simulink model "zzz"  (R2016b)
settings: Solver=ode4  StartTime=0.0  StopTime=inf  FixedStep=0.002  RelTol=1e-3  EnableMultiTasking=on
undefined symbols (not defined in the file or in its folder): bit, mdaadlink6208, sigbuilder_block, Standard
libraries: slrtlib x19, simulink x15, slrtsoftinglib x11
(part 2 of 3)

== system zzz/guangaiquxian ==
  In1 : Inport
  Chart1 : Stateflow chart  TreatAsAtomicUnit=on
  Display : Display
  Fcn : Fcn  Expr=(3.76012963313985e-12)*u^16-(3.44037229998304e-10)*u^15+(1.39996774652558e-08)*u^14-(3.34309394387153e-07)*u^13+(5.21860519506510e-06)*u^12-(5.63398801585665e-05)*u^11+0.000435175092700704*u^10-0.00244274561068785*u^9+0.00982136561852038*u^8-0.0269377658736148*u^7+0.0514170009108526*u^6-0.103245210636221*u^5+0.431283025667506*u^4-2.79148222601809*u^3+0.0172306812740196*u^2-0.00241932536131526*u+600.000082443648
  Saturation : Saturate  UpperLimit=12  LowerLimit=0
  Saturation1 : Saturate  UpperLimit=600  LowerLimit=20
  Out1 : Outport
  wires:
  In1/1 -> Chart1/1(a)
  Chart1/1(t) -> Saturation/1
  Saturation/1 -> Fcn/1
  Fcn/1 -> Saturation1/1
  Saturation1/1 -> Display/1, Out1/1

== system zzz/jinjichuli ==
  tiaoshi : Inport
  fa : Inport  Port=2
  jiting : Inport  Port=3
  Enable : EnablePort  StatesWhenEnabling=reset
  Demux : Demux  Outputs=16
  Mux : Mux  Inputs=16
  jinjichuli : Stateflow chart  TreatAsAtomicUnit=on
  Out1 : Outport
  wires:
  tiaoshi/1 -> jinjichuli/1(tiaoshi)
  fa/1 -> Demux/1
  Demux/1 -> jinjichuli/2(fa11_1)
  Demux/2 -> jinjichuli/3(fa11_2)
  Demux/3 -> jinjichuli/4(fa11_5)
  Demux/4 -> jinjichuli/5(fa20)
  Demux/5 -> jinjichuli/6(fa16_1)
  Demux/6 -> jinjichuli/7(fa3)
  Demux/7 -> jinjichuli/8(fa21)
  Demux/12 -> jinjichuli/13(fa18_1)
  Demux/13 -> jinjichuli/14(fa18_2)
  jiting/1 -> jinjichuli/18(jiting)
  Demux/14 -> jinjichuli/15(fa18_3)
  Demux/15 -> jinjichuli/16(fa18_4)
  Demux/16 -> jinjichuli/17(fa_kgg)
  jinjichuli/1(diancifa11_1) -> Mux/1
  jinjichuli/2(diancifa11_2) -> Mux/2
  jinjichuli/3(diancifa11_5) -> Mux/3
  jinjichuli/4(diancifa20) -> Mux/4
  jinjichuli/5(diancifa16_1) -> Mux/5
  jinjichuli/6(diancifa3) -> Mux/6
  jinjichuli/7(diancifa21) -> Mux/7
  jinjichuli/12(bililiuliangfa18_1) -> Mux/12
  jinjichuli/13(bililiuliangfa18_2) -> Mux/13
  jinjichuli/14(bililiuliangfa18_3) -> Mux/14
  jinjichuli/15(bililiuliangfa18_4) -> Mux/15
  jinjichuli/16(kaiguangaifa) -> Mux/16
  Mux/1 -> Out1/1
  Demux/8 -> jinjichuli/9(suodingmingling)
  Demux/9 -> jinjichuli/10(jiesuomingling)
  Demux/10 -> jinjichuli/11(xuansongmingling)
  Demux/11 -> jinjichuli/12(xuanjinmingling)
  jinjichuli/8(suoding) -> Mux/8
  jinjichuli/9(jiesuo) -> Mux/9
  jinjichuli/10(xuansong) -> Mux/10
  jinjichuli/11(xuanjin) -> Mux/11

== system zzz/kaigaiquxian ==
  In1 : Inport
  Chart : Stateflow chart  TreatAsAtomicUnit=on
  Display : Display
  Fcn : Fcn  Expr=(3.76012794303783e-12)*u^16-(3.77787151438439e-10)*u^15+(1.70366716702520e-08)*u^14-(4.53918294904343e-07)*u^13+(7.91595568148143e-06)*u^12-(9.46991801150381e-05)*u^11+0.000795158956924619*u^10-0.00475883386986616*u^9+0.0207391801532158*u^8-0.0673081776269616*u^7+0.155366359479885*u^6-0.201490925155371*u^5-0.0768516231318135*u^4+2.18034933328387*u^3+0.0584293012534094*u^2-0.00654372848246011*u+20.0002376678902
  Saturation : Saturate  UpperLimit=12  LowerLimit=0
  Saturation1 : Saturate  UpperLimit=600  LowerLimit=20
  Out1 : Outport
  wires:
  In1/1 -> Chart/1(a)
  Saturation/1 -> Fcn/1
  Chart/1(t) -> Saturation/1
  Fcn/1 -> Saturation1/1
  Saturation1/1 -> Display/1, Out1/1

== system zzz/tiaoshifa ==
  Mux3 : Mux  Inputs=16
  fa11_1 : Constant  Value=0
      settings: OpenFcn=|
      | if get_param(gcb,'value')=='1',
      | set_param(gcb,'value','0');
      | else
      | set_param(gcb,'value','1');end
  fa11_2 : Constant  Value=0
      settings: OpenFcn=|
      | if get_param(gcb,'value')=='1',
      | set_param(gcb,'value','0');
      | else
      | set_param(gcb,'value','1');end
  fa11_5 : Constant  Value=0
      settings: OpenFcn=|
      | if get_param(gcb,'value')=='1',
      | set_param(gcb,'value','0');
      | else
      | set_param(gcb,'value','1');end
  fa16_1 : Constant  Value=0
      settings: OpenFcn=|
      | if get_param(gcb,'value')=='1',
      | set_param(gcb,'value','0');
      | else
      | set_param(gcb,'value','1');end
  fa18_{1..4} (4 alike) : Constant  Value=0
  fa20 : Constant  Value=0
      settings: OpenFcn=|
      | if get_param(gcb,'value')=='1',
      | set_param(gcb,'value','0');
      | else
      | set_param(gcb,'value','1');end
  fa21 : Constant  Value=0
      settings: OpenFcn=|
      | if get_param(gcb,'value')=='1',
      | set_param(gcb,'value','0');
      | else
      | set_param(gcb,'value','1');end
  fa3 : Constant  Value=0
      settings: OpenFcn=|
      | if get_param(gcb,'value')=='1',
      | set_param(gcb,'value','0');
      | else
      | set_param(gcb,'value','1');end
  fa_kgg : Constant  Value=0
  jiesuomingling : Constant  Value=0
      settings: OpenFcn=|
      | if get_param(gcb,'value')=='1',
      | set_param(gcb,'value','0');
      | else
      | set_param(gcb,'value','1');end
  suodingmingling : Constant  Value=0
      settings: OpenFcn=|
      | if get_param(gcb,'value')=='1',
      | set_param(gcb,'value','0');
      | else
      | set_param(gcb,'value','1');end
  xuanjinmingling : Constant  Value=0
      settings: OpenFcn=|
      | if get_param(gcb,'value')=='1',
      | set_param(gcb,'value','0');
      | else
      | set_param(gcb,'value','1');end
  xuansongmingling : Constant  Value=0
      settings: OpenFcn=|
      | if get_param(gcb,'value')=='1',
      | set_param(gcb,'value','0');
      | else
      | set_param(gcb,'value','1');end
  Out1 : Outport
  wires:
  fa11_5/1 -> Mux3/3
  fa20/1 -> Mux3/4
  jiesuomingling/1 -> Mux3/11
  xuanjinmingling/1 -> Mux3/9
  fa_kgg/1 -> Mux3/16
  fa11_2/1 -> Mux3/2
  fa11_1/1 -> Mux3/1
  fa16_1/1 -> Mux3/5
  xuansongmingling/1 -> Mux3/8
  fa21/1 -> Mux3/7
  suodingmingling/1 -> Mux3/10
  fa3/1 -> Mux3/6
  Mux3/1 -> Out1/1
  fa18_1/1 -> Mux3/12
  fa18_2/1 -> Mux3/13
  fa18_3/1 -> Mux3/14
  fa18_4/1 -> Mux3/15

== system zzz/Subsystem2/husuo ==
  In1 : Inport
  In2 : Inport  Port=2
  Constant : Constant  Value=0
  Constant2 : Constant  Value=0
  Memory : Memory
  Memory1 : Memory
  Switch : Switch  Criteria=u2 > Threshold  Threshold=0.5
  Switch2 : Switch  Criteria=u2 > Threshold  Threshold=0.5
  Out1 : Outport
  Out2 : Outport  Port=2
  wires:
  Memory/1 -> Switch/2
  Memory1/1 -> Switch2/2
  In1/1 -> Switch/3
  In2/1 -> Switch2/3
  Constant2/1 -> Switch2/1
  Switch/1 -> Memory1/1, Out1/1
  Constant/1 -> Switch/1
  Switch2/1 -> Out2/1, Memory/1

== system zzz/Subsystem2/husuo1 ==
  In1 : Inport
  In2 : Inport  Port=2
  Constant : Constant  Value=0
  Constant2 : Constant  Value=0
  Memory : Memory
  Memory1 : Memory
  Switch : Switch  Criteria=u2 > Threshold  Threshold=0.5
  Switch2 : Switch  Criteria=u2 > Threshold  Threshold=0.5
  Out1 : Outport
  Out2 : Outport  Port=2
  wires:
  Switch2/1 -> Memory/1, Out2/1
  Constant/1 -> Switch/1
  Switch/1 -> Out1/1, Memory1/1
  Constant2/1 -> Switch2/1
  In2/1 -> Switch2/3
  In1/1 -> Switch/3
  Memory1/1 -> Switch2/2
  Memory/1 -> Switch/2

== system zzz/Subsystem2/husuo2 ==
  In1 : Inport
  In2 : Inport  Port=2
  Constant : Constant  Value=0
  Constant2 : Constant  Value=0
  Memory : Memory
  Memory1 : Memory
  Switch : Switch  Criteria=u2 > Threshold  Threshold=0.5
  Switch2 : Switch  Criteria=u2 > Threshold  Threshold=0.5
  Out1 : Outport
  Out2 : Outport  Port=2
  wires:
  Memory/1 -> Switch/2
  Memory1/1 -> Switch2/2
  In1/1 -> Switch/3
  In2/1 -> Switch2/3
  Constant2/1 -> Switch2/1
  Switch/1 -> Memory1/1, Out1/1
  Constant/1 -> Switch/1
  Switch2/1 -> Out2/1, Memory/1

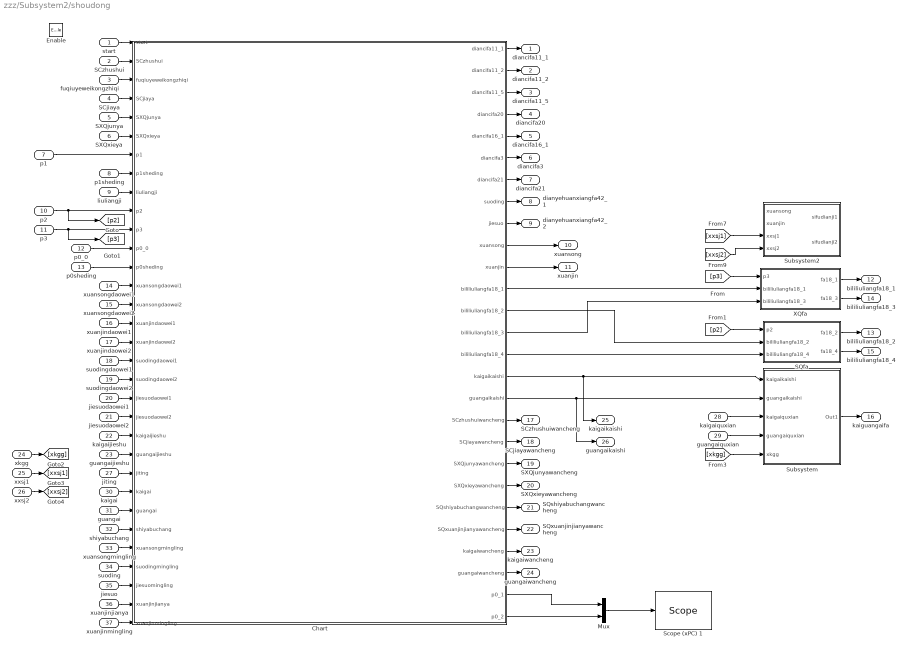
== system zzz/Subsystem2/shoudong ==
  start : Inport
  SCzhushui : Inport  Port=2
  fuqiuyeweikongzhiqi : Inport  Port=3
  SCjiaya : Inport  Port=4
  SXQjunya : Inport  Port=5
  SXQxieya : Inport  Port=6
  p1 : Inport  Port=7
  p1sheding : Inport  Port=8
  liuliangji : Inport  Port=9
  p2 : Inport  Port=10
  p3 : Inport  Port=11
  p0_0 : Inport  Port=12
  p0sheding : Inport  Port=13
  xuansongdaowei1 : Inport  Port=14
  xuansongdaowei2 : Inport  Port=15
  xuanjindaowei1 : Inport  Port=16
  xuanjindaowei2 : Inport  Port=17
  suodingdaowei1 : Inport  Port=18
  suodingdaowei2 : Inport  Port=19
  jiesuodaowei1 : Inport  Port=20
  jiesuodaowei2 : Inport  Port=21
  kaigaijieshu : Inport  Port=22
  guangaijieshu : Inport  Port=23
  xkgg : Inport  Port=24
  xxsj1 : Inport  Port=25
  xxsj2 : Inport  Port=26
  jiting : Inport  Port=27
  kaigaiquxian : Inport  Port=28
  guangaiquxian : Inport  Port=29
  kaigai : Inport  Port=30
  guangai : Inport  Port=31
  shiyabuchang : Inport  Port=32
  xuansongmingling : Inport  Port=33
  suoding : Inport  Port=34
  jiesuo : Inport  Port=35
  xuanjinjianya : Inport  Port=36
  xuanjinmingling : Inport  Port=37
  Enable : EnablePort
  Chart : Stateflow chart  TreatAsAtomicUnit=on
  Mux : Mux  Inputs=2
  SQfa : Subsystem
  Scope (xPC) 1 : slrtlib/Displays and Logging/Scope   scopeno=5  scopetype=Target  autostart=on  viewmode=Numerical  formatstr='%15.6f'  grid=on  ylimits=[0,0]  nosamples=250  noprepostsamples=0  interleave=1  triggermode=FreeRun  triggersignal=1  trigsignalfromport=off  triggerlevel=0.0  triggerslope=Either  triggerscope=1  triggersample=0  filename=data.dat  mode=Lazy  writesize=512  autorestart=off  dynamicfilemode=off  maxwritefilesize=512*1024^2
  Subsystem : Subsystem
  Subsystem2 : Subsystem
  XQfa : Subsystem
  diancifa11_1 : Outport
  diancifa11_2 : Outport  Port=2
  diancifa11_5 : Outport  Port=3
  diancifa20 : Outport  Port=4
  diancifa16_1 : Outport  Port=5
  diancifa3 : Outport  Port=6
  diancifa21 : Outport  Port=7
  dianyehuanxiangfa42_1 : Outport  Port=8
  dianyehuanxiangfa42_2 : Outport  Port=9
  xuansong : Outport  Port=10
  xuanjin : Outport  Port=11
  bililiuliangfa18_1 : Outport  Port=12
  bililiuliangfa18_2 : Outport  Port=13
  bililiuliangfa18_3 : Outport  Port=14
  bililiuliangfa18_4 : Outport  Port=15
  kaiguangaifa : Outport  Port=16
  SCzhushuiwancheng : Outport  Port=17
  SCjiayawancheng : Outport  Port=18
  SXQjunyawancheng : Outport  Port=19
  SXQxieyawancheng : Outport  Port=20
  SQshiyabuchangwancheng : Outport  Port=21
  SQxuanjinjianyawancheng : Outport  Port=22
  kaigaiwancheng : Outport  Port=23
  guangaiwancheng : Outport  Port=24
  kaigaikaishi : Outport  Port=25
  guangaikaishi : Outport  Port=26
  wires:
  jiting/1 -> Chart/24(jiting)
  xkgg/1 -> [xkgg]
  Chart/23(SQxuanjinjianyawancheng) -> SQxuanjinjianyawancheng/1
  Chart/22(SQshiyabuchangwancheng) -> SQshiyabuchangwancheng/1
  Chart/21(SXQxieyawancheng) -> SXQxieyawancheng/1
  Chart/20(SXQjunyawancheng) -> SXQjunyawancheng/1
  Chart/19(SCjiayawancheng) -> SCjiayawancheng/1
  Chart/18(SCzhushuiwancheng) -> SCzhushuiwancheng/1
  Chart/9(jiesuo) -> dianyehuanxiangfa42_2/1
  Chart/8(suoding) -> dianyehuanxiangfa42_1/1
  Chart/25(guangaiwancheng) -> guangaiwancheng/1
  guangaijieshu/1 -> Chart/23(guangaijieshu)
  Chart/24(kaigaiwancheng) -> kaigaiwancheng/1
  kaigaijieshu/1 -> Chart/22(kaigaijieshu)
  jiesuodaowei2/1 -> Chart/21(jiesuodaowei2)
  jiesuodaowei1/1 -> Chart/20(jiesuodaowei1)
  suodingdaowei2/1 -> Chart/19(suodingdaowei2)
  suodingdaowei1/1 -> Chart/18(suodingdaowei1)
  xuanjindaowei2/1 -> Chart/17(xuanjindaowei2)
  xuanjindaowei1/1 -> Chart/16(xuanjindaowei1)
  xuansongdaowei2/1 -> Chart/15(xuansongdaowei2)
  xuansongdaowei1/1 -> Chart/14(xuansongdaowei1)
  guangai/1 -> Chart/26(guangai)
  kaigai/1 -> Chart/25(kaigai)
  SQfa/2(fa18_4) -> bililiuliangfa18_4/1
  SQfa/1(fa18_2) -> bililiuliangfa18_2/1
  liuliangji/1 -> Chart/9(liuliangji)
  XQfa/2(fa18_3) -> bililiuliangfa18_3/1
  Chart/7(diancifa21) -> diancifa21/1
  XQfa/1(fa18_1) -> bililiuliangfa18_1/1
  Chart/6(diancifa3) -> diancifa3/1
  SXQxieya/1 -> Chart/6(SXQxieya)
  Chart/5(diancifa16_1) -> diancifa16_1/1
  SXQjunya/1 -> Chart/5(SXQjunya)
  Chart/4(diancifa20) -> diancifa20/1
  SCjiaya/1 -> Chart/4(SCjiaya)
  Chart/3(diancifa11_5) -> diancifa11_5/1
  fuqiuyeweikongzhiqi/1 -> Chart/3(fuqiuyeweikongzhiqi)
  Chart/2(diancifa11_2) -> diancifa11_2/1
  SCzhushui/1 -> Chart/2(SCzhushui)
  Chart/1(diancifa11_1) -> diancifa11_1/1
  start/1 -> Chart/1(start)
  p1/1 -> Chart/7(p1)
  [p2] -> SQfa/1(p2)
  [p3] -> XQfa/1(p3)
  p3/1 -> [p3], Chart/11(p3)
  p2/1 -> [p2], Chart/10(p2)
  p0_0/1 -> Chart/12(p0_0)
  p0sheding/1 -> Chart/13(p0sheding)
  p1sheding/1 -> Chart/8(p1sheding)
  Chart/15(bililiuliangfa18_4) -> SQfa/3(bililiuliangfa18_4)
  Chart/12(bililiuliangfa18_1) -> XQfa/2(bililiuliangfa18_1)
  Chart/13(bililiuliangfa18_2) -> SQfa/2(bililiuliangfa18_2)
  Chart/14(bililiuliangfa18_3) -> XQfa/3(bililiuliangfa18_3)
  shiyabuchang/1 -> Chart/27(shiyabuchang)
  xuansongmingling/1 -> Chart/28(xuansongmingling)
  suoding/1 -> Chart/29(suodingmingling)
  jiesuo/1 -> Chart/30(jiesuomingling)
  xuanjinjianya/1 -> Chart/31(xuanjinjianya)
  xuanjinmingling/1 -> Chart/32(xuanjinmingling)
  xxsj1/1 -> [xxsj1]
  xxsj2/1 -> [xxsj2]
  [xkgg] -> Subsystem/5(xkgg)
  Subsystem/1(Out1) -> kaiguangaifa/1
  [xxsj2] -> Subsystem2/4(xxsj2)
  [xxsj1] -> Subsystem2/3(xxsj1)
  Chart/10(xuansong) -> xuansong/1
  Chart/11(xuanjin) -> xuanjin/1
  Chart/26(p0_1) -> Mux/1
  Chart/27(p0_2) -> Mux/2
  Mux/1 -> Scope (xPC) 1/1
  Chart/16(kaigaikaishi) -> kaigaikaishi/1, Subsystem/1(kaigaikaishi)
  Chart/17(guangaikaishi) -> Subsystem/2(guangaikaishi), guangaikaishi/1
  guangaiquxian/1 -> Subsystem/4(guangaiquxian)
  kaigaiquxian/1 -> Subsystem/3(kaigaiquxian)

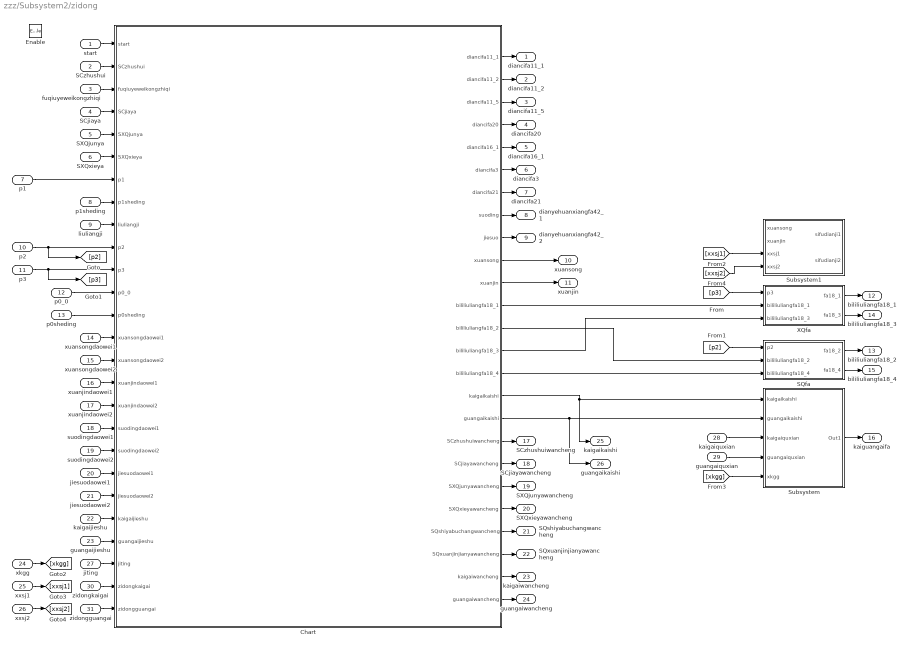
== system zzz/Subsystem2/zidong ==
  start : Inport
  SCzhushui : Inport  Port=2
  fuqiuyeweikongzhiqi : Inport  Port=3
  SCjiaya : Inport  Port=4
  SXQjunya : Inport  Port=5
  SXQxieya : Inport  Port=6
  p1 : Inport  Port=7
  p1sheding : Inport  Port=8
  liuliangji : Inport  Port=9
  p2 : Inport  Port=10
  p3 : Inport  Port=11
  p0_0 : Inport  Port=12
  p0sheding : Inport  Port=13
  xuansongdaowei1 : Inport  Port=14
  xuansongdaowei2 : Inport  Port=15
  xuanjindaowei1 : Inport  Port=16
  xuanjindaowei2 : Inport  Port=17
  suodingdaowei1 : Inport  Port=18
  suodingdaowei2 : Inport  Port=19
  jiesuodaowei1 : Inport  Port=20
  jiesuodaowei2 : Inport  Port=21
  kaigaijieshu : Inport  Port=22
  guangaijieshu : Inport  Port=23
  xkgg : Inport  Port=24
  xxsj1 : Inport  Port=25
  xxsj2 : Inport  Port=26
  jiting : Inport  Port=27
  kaigaiquxian : Inport  Port=28
  guangaiquxian : Inport  Port=29
  zidongkaigai : Inport  Port=30
  zidongguangai : Inport  Port=31
  Enable : EnablePort
  Chart : Stateflow chart  TreatAsAtomicUnit=on
  SQfa : Subsystem
  Subsystem : Subsystem
  Subsystem1 : Subsystem
  XQfa : Subsystem
  diancifa11_1 : Outport
  diancifa11_2 : Outport  Port=2
  diancifa11_5 : Outport  Port=3
  diancifa20 : Outport  Port=4
  diancifa16_1 : Outport  Port=5
  diancifa3 : Outport  Port=6
  diancifa21 : Outport  Port=7
  dianyehuanxiangfa42_1 : Outport  Port=8
  dianyehuanxiangfa42_2 : Outport  Port=9
  xuansong : Outport  Port=10
  xuanjin : Outport  Port=11
  bililiuliangfa18_1 : Outport  Port=12
  bililiuliangfa18_2 : Outport  Port=13
  bililiuliangfa18_3 : Outport  Port=14
  bililiuliangfa18_4 : Outport  Port=15
  kaiguangaifa : Outport  Port=16
  SCzhushuiwancheng : Outport  Port=17
  SCjiayawancheng : Outport  Port=18
  SXQjunyawancheng : Outport  Port=19
  SXQxieyawancheng : Outport  Port=20
  SQshiyabuchangwancheng : Outport  Port=21
  SQxuanjinjianyawancheng : Outport  Port=22
  kaigaiwancheng : Outport  Port=23
  guangaiwancheng : Outport  Port=24
  kaigaikaishi : Outport  Port=25
  guangaikaishi : Outport  Port=26
  wires:
  Chart/14(bililiuliangfa18_3) -> XQfa/3(bililiuliangfa18_3)
  Chart/13(bililiuliangfa18_2) -> SQfa/2(bililiuliangfa18_2)
  Chart/12(bililiuliangfa18_1) -> XQfa/2(bililiuliangfa18_1)
  Chart/15(bililiuliangfa18_4) -> SQfa/3(bililiuliangfa18_4)
  p1sheding/1 -> Chart/8(p1sheding)
  p0sheding/1 -> Chart/13(p0sheding)
  p0_0/1 -> Chart/12(p0_0)
  p2/1 -> Chart/10(p2), [p2]
  p3/1 -> Chart/11(p3), [p3]
  [p3] -> XQfa/1(p3)
  [p2] -> SQfa/1(p2)
  p1/1 -> Chart/7(p1)
  start/1 -> Chart/1(start)
  Chart/1(diancifa11_1) -> diancifa11_1/1
  SCzhushui/1 -> Chart/2(SCzhushui)
  Chart/2(diancifa11_2) -> diancifa11_2/1
  fuqiuyeweikongzhiqi/1 -> Chart/3(fuqiuyeweikongzhiqi)
  Chart/3(diancifa11_5) -> diancifa11_5/1
  SCjiaya/1 -> Chart/4(SCjiaya)
  Chart/4(diancifa20) -> diancifa20/1
  SXQjunya/1 -> Chart/5(SXQjunya)
  Chart/5(diancifa16_1) -> diancifa16_1/1
  SXQxieya/1 -> Chart/6(SXQxieya)
  Chart/6(diancifa3) -> diancifa3/1
  XQfa/1(fa18_1) -> bililiuliangfa18_1/1
  Chart/7(diancifa21) -> diancifa21/1
  XQfa/2(fa18_3) -> bililiuliangfa18_3/1
  liuliangji/1 -> Chart/9(liuliangji)
  SQfa/1(fa18_2) -> bililiuliangfa18_2/1
  SQfa/2(fa18_4) -> bililiuliangfa18_4/1
  zidongkaigai/1 -> Chart/25(zidongkaigai)
  zidongguangai/1 -> Chart/26(zidongguangai)
  xuansongdaowei1/1 -> Chart/14(xuansongdaowei1)
  xuansongdaowei2/1 -> Chart/15(xuansongdaowei2)
  xuanjindaowei1/1 -> Chart/16(xuanjindaowei1)
  xuanjindaowei2/1 -> Chart/17(xuanjindaowei2)
  suodingdaowei1/1 -> Chart/18(suodingdaowei1)
  suodingdaowei2/1 -> Chart/19(suodingdaowei2)
  jiesuodaowei1/1 -> Chart/20(jiesuodaowei1)
  jiesuodaowei2/1 -> Chart/21(jiesuodaowei2)
  kaigaijieshu/1 -> Chart/22(kaigaijieshu)
  Chart/24(kaigaiwancheng) -> kaigaiwancheng/1
  guangaijieshu/1 -> Chart/23(guangaijieshu)
  Chart/25(guangaiwancheng) -> guangaiwancheng/1
  Chart/8(suoding) -> dianyehuanxiangfa42_1/1
  Chart/9(jiesuo) -> dianyehuanxiangfa42_2/1
  Chart/18(SCzhushuiwancheng) -> SCzhushuiwancheng/1
  Chart/19(SCjiayawancheng) -> SCjiayawancheng/1
  Chart/20(SXQjunyawancheng) -> SXQjunyawancheng/1
  Chart/21(SXQxieyawancheng) -> SXQxieyawancheng/1
  Chart/22(SQshiyabuchangwancheng) -> SQshiyabuchangwancheng/1
  Chart/23(SQxuanjinjianyawancheng) -> SQxuanjinjianyawancheng/1
  xkgg/1 -> [xkgg]
  jiting/1 -> Chart/24(jiting)
  xxsj1/1 -> [xxsj1]
  xxsj2/1 -> [xxsj2]
  Chart/16(kaigaikaishi) -> kaigaikaishi/1, Subsystem/1(kaigaikaishi)
  Chart/17(guangaikaishi) -> guangaikaishi/1, Subsystem/2(guangaikaishi)
  [xkgg] -> Subsystem/5(xkgg)
  Subsystem/1(Out1) -> kaiguangaifa/1
  [xxsj2] -> Subsystem1/4(xxsj2)
  [xxsj1] -> Subsystem1/3(xxsj1)
  Chart/10(xuansong) -> xuansong/1
  Chart/11(xuanjin) -> xuanjin/1
  kaigaiquxian/1 -> Subsystem/3(kaigaiquxian)
  guangaiquxian/1 -> Subsystem/4(guangaiquxian)

== system zzz/chuanganqi/yalishangxiaxian ==
  In1 : Inport
  Compare To Constant{,2,4,6,8,10} (6 alike) : simulink/Logic and Bit Operations/Compare To Constant  relop=<=  const=0.1  OutDataTypeStr=boolean
  Compare To Constant{1,3,5,7,9,11} (6 alike) : simulink/Logic and Bit Operations/Compare To Constant  relop=>=  const=0.33  OutDataTypeStr=boolean
  Demux5 : Demux  Outputs=6
  Logical Operator : Logic  Operator=OR  Inputs=12  AllPortsSameDT=off  OutDataTypeStr=boolean
  Out1 : Outport
  wires:
  Demux5/2 -> Compare To Constant3/1, Compare To Constant2/1
  Demux5/6 -> Compare To Constant11/1, Compare To Constant10/1
  Compare To Constant/1 -> Logical Operator/1
  Demux5/4 -> Compare To Constant7/1, Compare To Constant6/1
  Compare To Constant8/1 -> Logical Operator/9
  Compare To Constant9/1 -> Logical Operator/10
  Compare To Constant4/1 -> Logical Operator/5
  Compare To Constant5/1 -> Logical Operator/6
  Compare To Constant2/1 -> Logical Operator/3
  Compare To Constant3/1 -> Logical Operator/4
  Compare To Constant6/1 -> Logical Operator/7
  Compare To Constant7/1 -> Logical Operator/8
  Compare To Constant11/1 -> Logical Operator/12
  Compare To Constant10/1 -> Logical Operator/11
  Demux5/3 -> Compare To Constant5/1, Compare To Constant4/1
  Demux5/1 -> Compare To Constant1/1, Compare To Constant/1
  Demux5/5 -> Compare To Constant9/1, Compare To Constant8/1
  In1/1 -> Demux5/1
  Compare To Constant1/1 -> Logical Operator/2
  Logical Operator/1 -> Out1/1

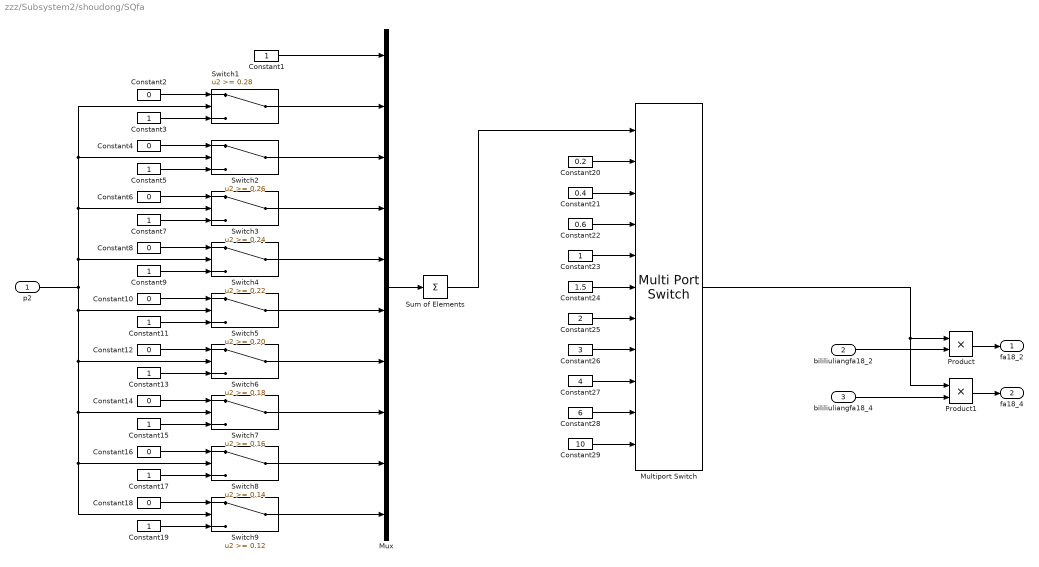
== system zzz/Subsystem2/shoudong/SQfa ==
  p2 : Inport
  bililiuliangfa18_2 : Inport  Port=2
  bililiuliangfa18_4 : Inport  Port=3
  Constant{1,3,5,7,9,11,13,15,17,19,23} (11 alike) : Constant
  Constant{2,4,6,8,10,12,14,16,18} (9 alike) : Constant  Value=0
  Constant20 : Constant  Value=0.2
  Constant21 : Constant  Value=0.4
  Constant22 : Constant  Value=0.6
  Constant24 : Constant  Value=1.5
  Constant25 : Constant  Value=2
  Constant26 : Constant  Value=3
  Constant27 : Constant  Value=4
  Constant28 : Constant  Value=6
  Constant29 : Constant  Value=10
  Multiport Switch : MultiPortSwitch  Inputs=10
  Mux : Mux  Inputs=10
  Product : Product  RndMeth=Zero
  Product1 : Product  RndMeth=Zero
  Sum of Elements : Sum  Inputs=+
  Switch1 : Switch  Threshold=0.28
  Switch2 : Switch  Threshold=0.26
  Switch3 : Switch  Threshold=0.24
  Switch4 : Switch  Threshold=0.22
  Switch5 : Switch  Threshold=0.20
  Switch6 : Switch  Threshold=0.18
  Switch7 : Switch  Threshold=0.16
  Switch8 : Switch  Threshold=0.14
  Switch9 : Switch  Threshold=0.12
  fa18_2 : Outport
  fa18_4 : Outport  Port=2
  wires:
  Constant2/1 -> Switch1/1
  Constant3/1 -> Switch1/3
  Constant4/1 -> Switch2/1
  Constant5/1 -> Switch2/3
  Constant6/1 -> Switch3/1
  Constant7/1 -> Switch3/3
  Constant8/1 -> Switch4/1
  Constant9/1 -> Switch4/3
  Constant10/1 -> Switch5/1
  Constant11/1 -> Switch5/3
  Constant12/1 -> Switch6/1
  Constant13/1 -> Switch6/3
  Constant14/1 -> Switch7/1
  Constant15/1 -> Switch7/3
  p2/1 -> Switch1/2, Switch2/2, Switch3/2, Switch4/2, Switch6/2, Switch7/2, Switch8/2, Switch9/2, Switch5/2
  Mux/1 -> Sum of Elements/1
  Sum of Elements/1 -> Multiport Switch/1
  Constant1/1 -> Mux/1
  Switch1/1 -> Mux/2
  Switch2/1 -> Mux/3
  Switch3/1 -> Mux/4
  Switch4/1 -> Mux/5
  Switch5/1 -> Mux/6
  Switch6/1 -> Mux/7
  Switch7/1 -> Mux/8
  Switch8/1 -> Mux/9
  Switch9/1 -> Mux/10
  Constant16/1 -> Switch8/1
  Constant17/1 -> Switch8/3
  Constant18/1 -> Switch9/1
  Constant19/1 -> Switch9/3
  Multiport Switch/1 -> Product/1, Product1/1
  Constant20/1 -> Multiport Switch/2
  Constant21/1 -> Multiport Switch/3
  Constant22/1 -> Multiport Switch/4
  Constant23/1 -> Multiport Switch/5
  Constant24/1 -> Multiport Switch/6
  Constant25/1 -> Multiport Switch/7
  Constant26/1 -> Multiport Switch/8
  Constant27/1 -> Multiport Switch/9
  Constant28/1 -> Multiport Switch/10
  Constant29/1 -> Multiport Switch/11
  bililiuliangfa18_2/1 -> Product/2
  bililiuliangfa18_4/1 -> Product1/2
  Product/1 -> fa18_2/1
  Product1/1 -> fa18_4/1

== system zzz/Subsystem2/shoudong/Subsystem ==
  kaigaikaishi : Inport
  guangaikaishi : Inport  Port=2
  kaigaiquxian : Inport  Port=3
  guangaiquxian : Inport  Port=4
  xkgg : Inport  Port=5
  Add1 : Sum
  Constant : Constant  Value=2
  Constant1 : Constant  Value=-0.05
  Display{,1..3} (4 alike) : Display
  Gain : Gain  Gain=0.1
  Gain1 : Gain  Gain=0.1
  Multiport Switch : MultiPortSwitch
  Product : Product
  Sum : Sum  Inputs=|+-
  Sum1 : Sum  Inputs=|+-
  Out1 : Outport
  wires:
  guangaikaishi/1 -> Product/1
  Constant/1 -> Product/2
  kaigaikaishi/1 -> Add1/1
  Product/1 -> Add1/2
  Add1/1 -> Multiport Switch/1
  Multiport Switch/1 -> Display2/1, Out1/1
  Sum/1 -> Gain/1
  Gain/1 -> Multiport Switch/2, Display1/1
  Sum1/1 -> Gain1/1
  Gain1/1 -> Display/1, Multiport Switch/3
  Constant1/1 -> Multiport Switch/4
  xkgg/1 -> Display3/1, Sum1/2, Sum/2
  kaigaiquxian/1 -> Sum/1
  guangaiquxian/1 -> Sum1/1

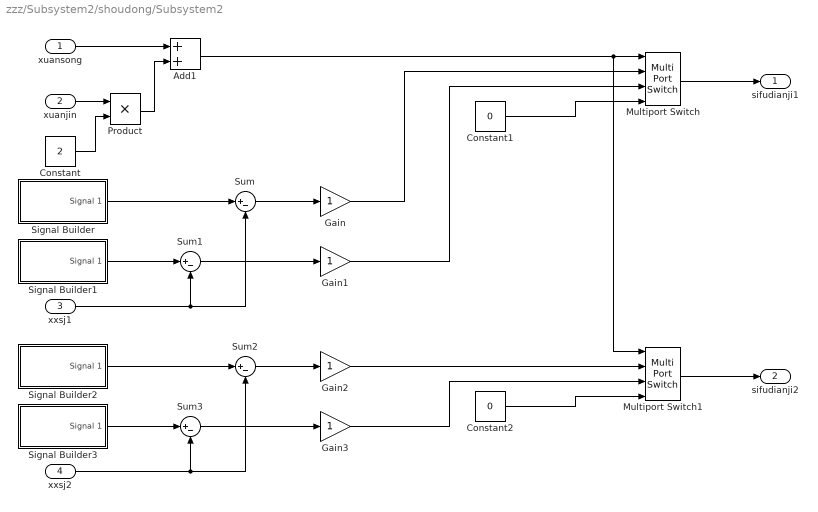
== system zzz/Subsystem2/shoudong/Subsystem2 ==
  xuansong : Inport
  xuanjin : Inport  Port=2
  xxsj1 : Inport  Port=3
  xxsj2 : Inport  Port=4
  Add1 : Sum
  Constant : Constant  Value=2
  Constant1 : Constant  Value=0
  Constant2 : Constant  Value=0
  Gain{,1..3} (4 alike) : Gain
  Multiport Switch : MultiPortSwitch
  Multiport Switch1 : MultiPortSwitch
  Product : Product
  Signal Builder : Subsystem  Tag=STV Subsys  LoadFcn=sigbuilder_block('load');  StartFcn=sigbuilder_block('start');  StopFcn=sigbuilder_block('stop');  ClipboardFcn=sigbuilder_block('clipboard');  mask(Sigbuilder block){tuvar=[0:10]}
      mask help: Simulink:masks:SigbuilderBlock_MD
      mask init:
      | if ~strcmp(get_param(bdroot(gcbh),'SimulationStatus'),'stopped') tuvar = sigbuilder_block('maskInit'); end
      settings: CopyFcn=sigbuilder_block('copy');  DeleteFcn=sigbuilder_block('delete');  ModelCloseFcn=sigbuilder_block('modelClose');  PreSaveFcn=sigbuilder_block('preSave');  PauseFcn=sigbuilder_block('pause');  ContinueFcn=sigbuilder_block('continue');  NameChangeFcn=sigbuilder_block('namechange');  OpenFcn=sigbuilder_block('open',[437.6 199.2 550.4 400 ]);  CloseFcn=sigbuilder_block('close');
      mask Display: plot(0, 0, 100, 100,[2, 2, 32, 32, 2], [68, 8, 8, 68, 68],[32, 2], [38, 38], [32, 19, 2],[53, 60, 44], [32, 17, 17, 2],[16, 16, 31, 31]);txt = getActiveGroup(gcbh);text(2, 100, txt,'verticalAlignment', 'top');
  Signal Builder1 : Subsystem  Tag=STV Subsys  LoadFcn=sigbuilder_block('load');  StartFcn=sigbuilder_block('start');  StopFcn=sigbuilder_block('stop');  ClipboardFcn=sigbuilder_block('clipboard');  mask(Sigbuilder block){tuvar=[0:10]}
      mask help: Simulink:masks:SigbuilderBlock_MD
      mask init:
      | if ~strcmp(get_param(bdroot(gcbh),'SimulationStatus'),'stopped') tuvar = sigbuilder_block('maskInit'); end
      settings: CopyFcn=sigbuilder_block('copy');  DeleteFcn=sigbuilder_block('delete');  ModelCloseFcn=sigbuilder_block('modelClose');  PreSaveFcn=sigbuilder_block('preSave');  PauseFcn=sigbuilder_block('pause');  ContinueFcn=sigbuilder_block('continue');  NameChangeFcn=sigbuilder_block('namechange');  OpenFcn=sigbuilder_block('open',[437.6 199.2 550.4 400 ]);  CloseFcn=sigbuilder_block('close');
      mask Display: plot(0, 0, 100, 100,[2, 2, 32, 32, 2], [68, 8, 8, 68, 68],[32, 2], [38, 38], [32, 19, 2],[53, 60, 44], [32, 17, 17, 2],[16, 16, 31, 31]);txt = getActiveGroup(gcbh);text(2, 100, txt,'verticalAlignment', 'top');
  Signal Builder2 : Subsystem  Tag=STV Subsys  LoadFcn=sigbuilder_block('load');  StartFcn=sigbuilder_block('start');  StopFcn=sigbuilder_block('stop');  ClipboardFcn=sigbuilder_block('clipboard');  mask(Sigbuilder block){tuvar=[0:10]}
      mask help: Simulink:masks:SigbuilderBlock_MD
      mask init:
      | if ~strcmp(get_param(bdroot(gcbh),'SimulationStatus'),'stopped') tuvar = sigbuilder_block('maskInit'); end
      settings: CopyFcn=sigbuilder_block('copy');  DeleteFcn=sigbuilder_block('delete');  ModelCloseFcn=sigbuilder_block('modelClose');  PreSaveFcn=sigbuilder_block('preSave');  PauseFcn=sigbuilder_block('pause');  ContinueFcn=sigbuilder_block('continue');  NameChangeFcn=sigbuilder_block('namechange');  OpenFcn=sigbuilder_block('open',[437.6 199.2 550.4 400 ]);  CloseFcn=sigbuilder_block('close');
      mask Display: plot(0, 0, 100, 100,[2, 2, 32, 32, 2], [68, 8, 8, 68, 68],[32, 2], [38, 38], [32, 19, 2],[53, 60, 44], [32, 17, 17, 2],[16, 16, 31, 31]);txt = getActiveGroup(gcbh);text(2, 100, txt,'verticalAlignment', 'top');
  Signal Builder3 : Subsystem  Tag=STV Subsys  LoadFcn=sigbuilder_block('load');  StartFcn=sigbuilder_block('start');  StopFcn=sigbuilder_block('stop');  ClipboardFcn=sigbuilder_block('clipboard');  mask(Sigbuilder block){tuvar=[0:10]}
      mask help: Simulink:masks:SigbuilderBlock_MD
      mask init:
      | if ~strcmp(get_param(bdroot(gcbh),'SimulationStatus'),'stopped') tuvar = sigbuilder_block('maskInit'); end
      settings: CopyFcn=sigbuilder_block('copy');  DeleteFcn=sigbuilder_block('delete');  ModelCloseFcn=sigbuilder_block('modelClose');  PreSaveFcn=sigbuilder_block('preSave');  PauseFcn=sigbuilder_block('pause');  ContinueFcn=sigbuilder_block('continue');  NameChangeFcn=sigbuilder_block('namechange');  OpenFcn=sigbuilder_block('open',[437.6 199.2 550.4 400 ]);  CloseFcn=sigbuilder_block('close');
      mask Display: plot(0, 0, 100, 100,[2, 2, 32, 32, 2], [68, 8, 8, 68, 68],[32, 2], [38, 38], [32, 19, 2],[53, 60, 44], [32, 17, 17, 2],[16, 16, 31, 31]);txt = getActiveGroup(gcbh);text(2, 100, txt,'verticalAlignment', 'top');
  Sum{,1..3} (4 alike) : Sum  Inputs=|+-
  sifudianji1 : Outport
  sifudianji2 : Outport  Port=2
  wires:
  Constant1/1 -> Multiport Switch/4
  Gain1/1 -> Multiport Switch/3
  Sum1/1 -> Gain1/1
  Signal Builder1/1(Signal 1) -> Sum1/1
  Gain/1 -> Multiport Switch/2
  Sum/1 -> Gain/1
  xxsj1/1 -> Sum/2, Sum1/2
  Signal Builder/1(Signal 1) -> Sum/1
  Multiport Switch/1 -> sifudianji1/1
  Add1/1 -> Multiport Switch1/1, Multiport Switch/1
  Product/1 -> Add1/2
  xuansong/1 -> Add1/1
  Constant/1 -> Product/2
  xuanjin/1 -> Product/1
  Multiport Switch1/1 -> sifudianji2/1
  Signal Builder2/1(Signal 1) -> Sum2/1
  xxsj2/1 -> Sum2/2, Sum3/2
  Sum2/1 -> Gain2/1
  Gain2/1 -> Multiport Switch1/2
  Signal Builder3/1(Signal 1) -> Sum3/1
  Sum3/1 -> Gain3/1
  Gain3/1 -> Multiport Switch1/3
  Constant2/1 -> Multiport Switch1/4

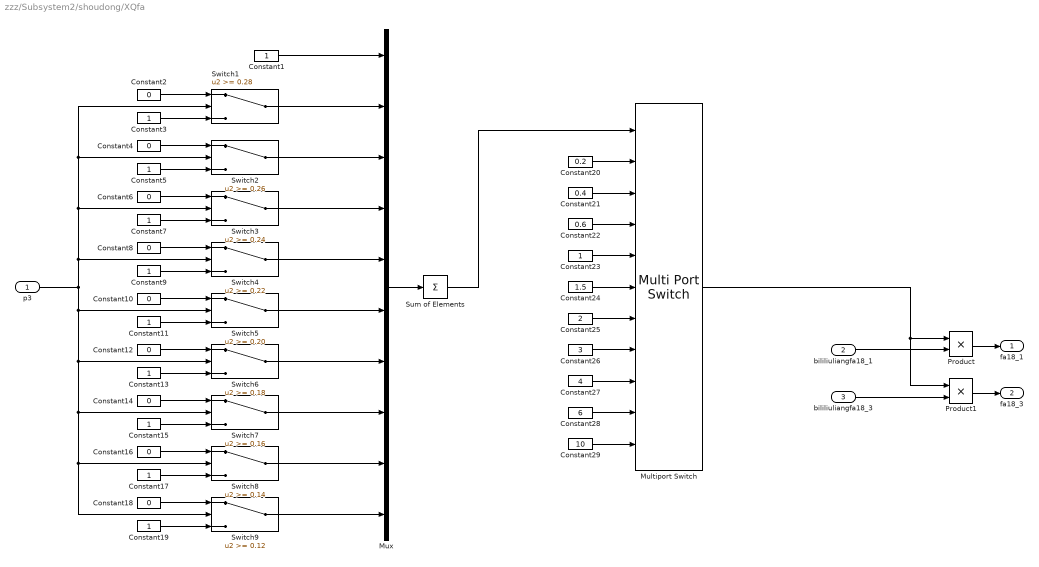
== system zzz/Subsystem2/shoudong/XQfa ==
  p3 : Inport
  bililiuliangfa18_1 : Inport  Port=2
  bililiuliangfa18_3 : Inport  Port=3
  Constant{1,3,5,7,9,11,13,15,17,19,23} (11 alike) : Constant
  Constant{2,4,6,8,10,12,14,16,18} (9 alike) : Constant  Value=0
  Constant20 : Constant  Value=0.2
  Constant21 : Constant  Value=0.4
  Constant22 : Constant  Value=0.6
  Constant24 : Constant  Value=1.5
  Constant25 : Constant  Value=2
  Constant26 : Constant  Value=3
  Constant27 : Constant  Value=4
  Constant28 : Constant  Value=6
  Constant29 : Constant  Value=10
  Multiport Switch : MultiPortSwitch  Inputs=10
  Mux : Mux  Inputs=10
  Product : Product  RndMeth=Zero
  Product1 : Product  RndMeth=Zero
  Sum of Elements : Sum  Inputs=+
  Switch1 : Switch  Threshold=0.28
  Switch2 : Switch  Threshold=0.26
  Switch3 : Switch  Threshold=0.24
  Switch4 : Switch  Threshold=0.22
  Switch5 : Switch  Threshold=0.20
  Switch6 : Switch  Threshold=0.18
  Switch7 : Switch  Threshold=0.16
  Switch8 : Switch  Threshold=0.14
  Switch9 : Switch  Threshold=0.12
  fa18_1 : Outport
  fa18_3 : Outport  Port=2
  wires:
  Product1/1 -> fa18_3/1
  Product/1 -> fa18_1/1
  bililiuliangfa18_3/1 -> Product1/2
  bililiuliangfa18_1/1 -> Product/2
  Constant29/1 -> Multiport Switch/11
  Constant28/1 -> Multiport Switch/10
  Constant27/1 -> Multiport Switch/9
  Constant26/1 -> Multiport Switch/8
  Constant25/1 -> Multiport Switch/7
  Constant24/1 -> Multiport Switch/6
  Constant23/1 -> Multiport Switch/5
  Constant22/1 -> Multiport Switch/4
  Constant21/1 -> Multiport Switch/3
  Constant20/1 -> Multiport Switch/2
  Multiport Switch/1 -> Product1/1, Product/1
  Constant19/1 -> Switch9/3
  Constant18/1 -> Switch9/1
  Constant17/1 -> Switch8/3
  Constant16/1 -> Switch8/1
  Switch9/1 -> Mux/10
  Switch8/1 -> Mux/9
  Switch7/1 -> Mux/8
  Switch6/1 -> Mux/7
  Switch5/1 -> Mux/6
  Switch4/1 -> Mux/5
  Switch3/1 -> Mux/4
  Switch2/1 -> Mux/3
  Switch1/1 -> Mux/2
  Constant1/1 -> Mux/1
  Sum of Elements/1 -> Multiport Switch/1
  Mux/1 -> Sum of Elements/1
  p3/1 -> Switch5/2, Switch9/2, Switch8/2, Switch7/2, Switch6/2, Switch4/2, Switch3/2, Switch2/2, Switch1/2
  Constant15/1 -> Switch7/3
  Constant14/1 -> Switch7/1
  Constant13/1 -> Switch6/3
  Constant12/1 -> Switch6/1
  Constant11/1 -> Switch5/3
  Constant10/1 -> Switch5/1
  Constant9/1 -> Switch4/3
  Constant8/1 -> Switch4/1
  Constant7/1 -> Switch3/3
  Constant6/1 -> Switch3/1
  Constant5/1 -> Switch2/3
  Constant4/1 -> Switch2/1
  Constant3/1 -> Switch1/3
  Constant2/1 -> Switch1/1

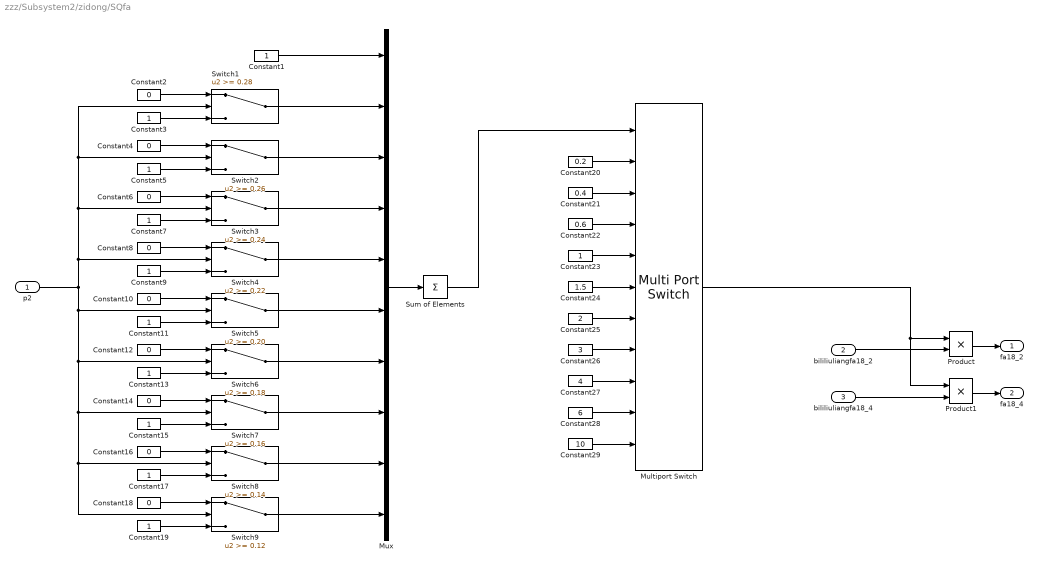
== system zzz/Subsystem2/zidong/SQfa ==
  p2 : Inport
  bililiuliangfa18_2 : Inport  Port=2
  bililiuliangfa18_4 : Inport  Port=3
  Constant{1,3,5,7,9,11,13,15,17,19,23} (11 alike) : Constant
  Constant{2,4,6,8,10,12,14,16,18} (9 alike) : Constant  Value=0
  Constant20 : Constant  Value=0.2
  Constant21 : Constant  Value=0.4
  Constant22 : Constant  Value=0.6
  Constant24 : Constant  Value=1.5
  Constant25 : Constant  Value=2
  Constant26 : Constant  Value=3
  Constant27 : Constant  Value=4
  Constant28 : Constant  Value=6
  Constant29 : Constant  Value=10
  Multiport Switch : MultiPortSwitch  Inputs=10
  Mux : Mux  Inputs=10
  Product : Product  RndMeth=Zero
  Product1 : Product  RndMeth=Zero
  Sum of Elements : Sum  Inputs=+
  Switch1 : Switch  Threshold=0.28
  Switch2 : Switch  Threshold=0.26
  Switch3 : Switch  Threshold=0.24
  Switch4 : Switch  Threshold=0.22
  Switch5 : Switch  Threshold=0.20
  Switch6 : Switch  Threshold=0.18
  Switch7 : Switch  Threshold=0.16
  Switch8 : Switch  Threshold=0.14
  Switch9 : Switch  Threshold=0.12
  fa18_2 : Outport
  fa18_4 : Outport  Port=2
  wires:
  Product1/1 -> fa18_4/1
  Product/1 -> fa18_2/1
  bililiuliangfa18_4/1 -> Product1/2
  bililiuliangfa18_2/1 -> Product/2
  Constant29/1 -> Multiport Switch/11
  Constant28/1 -> Multiport Switch/10
  Constant27/1 -> Multiport Switch/9
  Constant26/1 -> Multiport Switch/8
  Constant25/1 -> Multiport Switch/7
  Constant24/1 -> Multiport Switch/6
  Constant23/1 -> Multiport Switch/5
  Constant22/1 -> Multiport Switch/4
  Constant21/1 -> Multiport Switch/3
  Constant20/1 -> Multiport Switch/2
  Multiport Switch/1 -> Product1/1, Product/1
  Constant19/1 -> Switch9/3
  Constant18/1 -> Switch9/1
  Constant17/1 -> Switch8/3
  Constant16/1 -> Switch8/1
  Switch9/1 -> Mux/10
  Switch8/1 -> Mux/9
  Switch7/1 -> Mux/8
  Switch6/1 -> Mux/7
  Switch5/1 -> Mux/6
  Switch4/1 -> Mux/5
  Switch3/1 -> Mux/4
  Switch2/1 -> Mux/3
  Switch1/1 -> Mux/2
  Constant1/1 -> Mux/1
  Sum of Elements/1 -> Multiport Switch/1
  Mux/1 -> Sum of Elements/1
  p2/1 -> Switch5/2, Switch9/2, Switch8/2, Switch7/2, Switch6/2, Switch4/2, Switch3/2, Switch2/2, Switch1/2
  Constant15/1 -> Switch7/3
  Constant14/1 -> Switch7/1
  Constant13/1 -> Switch6/3
  Constant12/1 -> Switch6/1
  Constant11/1 -> Switch5/3
  Constant10/1 -> Switch5/1
  Constant9/1 -> Switch4/3
  Constant8/1 -> Switch4/1
  Constant7/1 -> Switch3/3
  Constant6/1 -> Switch3/1
  Constant5/1 -> Switch2/3
  Constant4/1 -> Switch2/1
  Constant3/1 -> Switch1/3
  Constant2/1 -> Switch1/1

== system zzz/Subsystem2/zidong/Subsystem ==
  kaigaikaishi : Inport
  guangaikaishi : Inport  Port=2
  kaigaiquxian : Inport  Port=3
  guangaiquxian : Inport  Port=4
  xkgg : Inport  Port=5
  Add1 : Sum
  Constant : Constant  Value=2
  Constant1 : Constant  Value=-0.05
  Display{,1..3} (4 alike) : Display
  Gain : Gain  Gain=0.1
  Gain1 : Gain  Gain=0.1
  Multiport Switch : MultiPortSwitch
  Product : Product
  Sum : Sum  Inputs=|+-
  Sum1 : Sum  Inputs=|+-
  Out1 : Outport
  wires:
  guangaikaishi/1 -> Product/1
  Constant/1 -> Product/2
  kaigaikaishi/1 -> Add1/1
  Product/1 -> Add1/2
  Add1/1 -> Multiport Switch/1
  Multiport Switch/1 -> Display2/1, Out1/1
  Sum/1 -> Gain/1
  Gain/1 -> Multiport Switch/2, Display1/1
  Sum1/1 -> Gain1/1
  Gain1/1 -> Display/1, Multiport Switch/3
  Constant1/1 -> Multiport Switch/4
  xkgg/1 -> Display3/1, Sum1/2, Sum/2
  kaigaiquxian/1 -> Sum/1
  guangaiquxian/1 -> Sum1/1

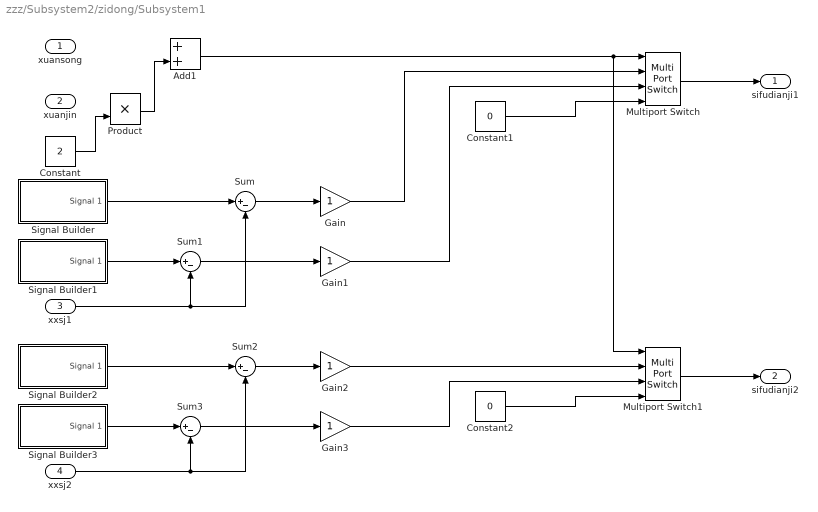
== system zzz/Subsystem2/zidong/Subsystem1 ==
  xuansong : Inport
  xuanjin : Inport  Port=2
  xxsj1 : Inport  Port=3
  xxsj2 : Inport  Port=4
  Add1 : Sum
  Constant : Constant  Value=2
  Constant1 : Constant  Value=0
  Constant2 : Constant  Value=0
  Gain{,1..3} (4 alike) : Gain
  Multiport Switch : MultiPortSwitch
  Multiport Switch1 : MultiPortSwitch
  Product : Product
  Signal Builder : Subsystem  Tag=STV Subsys  LoadFcn=sigbuilder_block('load');  StartFcn=sigbuilder_block('start');  StopFcn=sigbuilder_block('stop');  ClipboardFcn=sigbuilder_block('clipboard');  mask(Sigbuilder block){tuvar=[0:10]}
      mask help: Simulink:masks:SigbuilderBlock_MD
      mask init:
      | if ~strcmp(get_param(bdroot(gcbh),'SimulationStatus'),'stopped') tuvar = sigbuilder_block('maskInit'); end
      settings: CopyFcn=sigbuilder_block('copy');  DeleteFcn=sigbuilder_block('delete');  ModelCloseFcn=sigbuilder_block('modelClose');  PreSaveFcn=sigbuilder_block('preSave');  PauseFcn=sigbuilder_block('pause');  ContinueFcn=sigbuilder_block('continue');  NameChangeFcn=sigbuilder_block('namechange');  OpenFcn=sigbuilder_block('open',[437.6 199.2 550.4 400 ]);  CloseFcn=sigbuilder_block('close');
      mask Display: plot(0, 0, 100, 100,[2, 2, 32, 32, 2], [68, 8, 8, 68, 68],[32, 2], [38, 38], [32, 19, 2],[53, 60, 44], [32, 17, 17, 2],[16, 16, 31, 31]);txt = getActiveGroup(gcbh);text(2, 100, txt,'verticalAlignment', 'top');
  Signal Builder1 : Subsystem  Tag=STV Subsys  LoadFcn=sigbuilder_block('load');  StartFcn=sigbuilder_block('start');  StopFcn=sigbuilder_block('stop');  ClipboardFcn=sigbuilder_block('clipboard');  mask(Sigbuilder block){tuvar=[0:10]}
      mask help: Simulink:masks:SigbuilderBlock_MD
      mask init:
      | if ~strcmp(get_param(bdroot(gcbh),'SimulationStatus'),'stopped') tuvar = sigbuilder_block('maskInit'); end
      settings: CopyFcn=sigbuilder_block('copy');  DeleteFcn=sigbuilder_block('delete');  ModelCloseFcn=sigbuilder_block('modelClose');  PreSaveFcn=sigbuilder_block('preSave');  PauseFcn=sigbuilder_block('pause');  ContinueFcn=sigbuilder_block('continue');  NameChangeFcn=sigbuilder_block('namechange');  OpenFcn=sigbuilder_block('open',[437.6 199.2 550.4 400 ]);  CloseFcn=sigbuilder_block('close');
      mask Display: plot(0, 0, 100, 100,[2, 2, 32, 32, 2], [68, 8, 8, 68, 68],[32, 2], [38, 38], [32, 19, 2],[53, 60, 44], [32, 17, 17, 2],[16, 16, 31, 31]);txt = getActiveGroup(gcbh);text(2, 100, txt,'verticalAlignment', 'top');
  Signal Builder2 : Subsystem  Tag=STV Subsys  LoadFcn=sigbuilder_block('load');  StartFcn=sigbuilder_block('start');  StopFcn=sigbuilder_block('stop');  ClipboardFcn=sigbuilder_block('clipboard');  mask(Sigbuilder block){tuvar=[0:10]}
      mask help: Simulink:masks:SigbuilderBlock_MD
      mask init:
      | if ~strcmp(get_param(bdroot(gcbh),'SimulationStatus'),'stopped') tuvar = sigbuilder_block('maskInit'); end
      settings: CopyFcn=sigbuilder_block('copy');  DeleteFcn=sigbuilder_block('delete');  ModelCloseFcn=sigbuilder_block('modelClose');  PreSaveFcn=sigbuilder_block('preSave');  PauseFcn=sigbuilder_block('pause');  ContinueFcn=sigbuilder_block('continue');  NameChangeFcn=sigbuilder_block('namechange');  OpenFcn=sigbuilder_block('open',[437.6 199.2 550.4 400 ]);  CloseFcn=sigbuilder_block('close');
      mask Display: plot(0, 0, 100, 100,[2, 2, 32, 32, 2], [68, 8, 8, 68, 68],[32, 2], [38, 38], [32, 19, 2],[53, 60, 44], [32, 17, 17, 2],[16, 16, 31, 31]);txt = getActiveGroup(gcbh);text(2, 100, txt,'verticalAlignment', 'top');
  Signal Builder3 : Subsystem  Tag=STV Subsys  LoadFcn=sigbuilder_block('load');  StartFcn=sigbuilder_block('start');  StopFcn=sigbuilder_block('stop');  ClipboardFcn=sigbuilder_block('clipboard');  mask(Sigbuilder block){tuvar=[0:10]}
      mask help: Simulink:masks:SigbuilderBlock_MD
      mask init:
      | if ~strcmp(get_param(bdroot(gcbh),'SimulationStatus'),'stopped') tuvar = sigbuilder_block('maskInit'); end
      settings: CopyFcn=sigbuilder_block('copy');  DeleteFcn=sigbuilder_block('delete');  ModelCloseFcn=sigbuilder_block('modelClose');  PreSaveFcn=sigbuilder_block('preSave');  PauseFcn=sigbuilder_block('pause');  ContinueFcn=sigbuilder_block('continue');  NameChangeFcn=sigbuilder_block('namechange');  OpenFcn=sigbuilder_block('open',[437.6 199.2 550.4 400 ]);  CloseFcn=sigbuilder_block('close');
      mask Display: plot(0, 0, 100, 100,[2, 2, 32, 32, 2], [68, 8, 8, 68, 68],[32, 2], [38, 38], [32, 19, 2],[53, 60, 44], [32, 17, 17, 2],[16, 16, 31, 31]);txt = getActiveGroup(gcbh);text(2, 100, txt,'verticalAlignment', 'top');
  Sum{,1..3} (4 alike) : Sum  Inputs=|+-
  sifudianji1 : Outport
  sifudianji2 : Outport  Port=2
  wires:
  Constant1/1 -> Multiport Switch/4
  Gain1/1 -> Multiport Switch/3
  Sum1/1 -> Gain1/1
  Signal Builder1/1(Signal 1) -> Sum1/1
  Gain/1 -> Multiport Switch/2
  Sum/1 -> Gain/1
  xxsj1/1 -> Sum/2, Sum1/2
  Signal Builder/1(Signal 1) -> Sum/1
  Multiport Switch/1 -> sifudianji1/1
  Add1/1 -> Multiport Switch1/1, Multiport Switch/1
  Product/1 -> Add1/2
  Constant/1 -> Product/2
  Multiport Switch1/1 -> sifudianji2/1
  Signal Builder2/1(Signal 1) -> Sum2/1
  xxsj2/1 -> Sum2/2, Sum3/2
  Sum2/1 -> Gain2/1
  Gain2/1 -> Multiport Switch1/2
  Signal Builder3/1(Signal 1) -> Sum3/1
  Sum3/1 -> Gain3/1
  Gain3/1 -> Multiport Switch1/3
  Constant2/1 -> Multiport Switch1/4

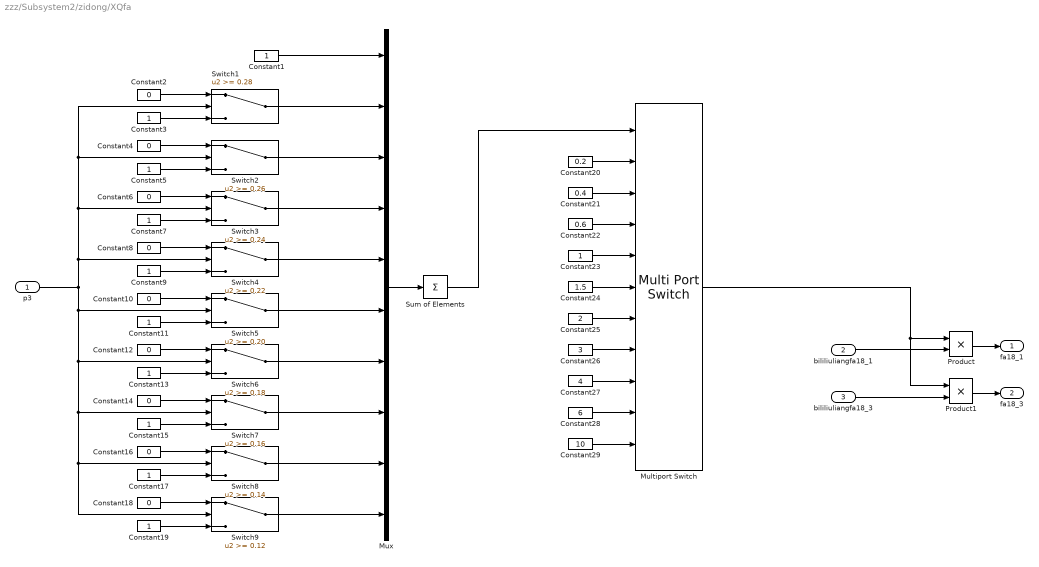
== system zzz/Subsystem2/zidong/XQfa ==
  p3 : Inport
  bililiuliangfa18_1 : Inport  Port=2
  bililiuliangfa18_3 : Inport  Port=3
  Constant{1,3,5,7,9,11,13,15,17,19,23} (11 alike) : Constant
  Constant{2,4,6,8,10,12,14,16,18} (9 alike) : Constant  Value=0
  Constant20 : Constant  Value=0.2
  Constant21 : Constant  Value=0.4
  Constant22 : Constant  Value=0.6
  Constant24 : Constant  Value=1.5
  Constant25 : Constant  Value=2
  Constant26 : Constant  Value=3
  Constant27 : Constant  Value=4
  Constant28 : Constant  Value=6
  Constant29 : Constant  Value=10
  Multiport Switch : MultiPortSwitch  Inputs=10
  Mux : Mux  Inputs=10
  Product : Product  RndMeth=Zero
  Product1 : Product  RndMeth=Zero
  Sum of Elements : Sum  Inputs=+
  Switch1 : Switch  Threshold=0.28
  Switch2 : Switch  Threshold=0.26
  Switch3 : Switch  Threshold=0.24
  Switch4 : Switch  Threshold=0.22
  Switch5 : Switch  Threshold=0.20
  Switch6 : Switch  Threshold=0.18
  Switch7 : Switch  Threshold=0.16
  Switch8 : Switch  Threshold=0.14
  Switch9 : Switch  Threshold=0.12
  fa18_1 : Outport
  fa18_3 : Outport  Port=2
  wires:
  Constant2/1 -> Switch1/1
  Constant3/1 -> Switch1/3
  Constant4/1 -> Switch2/1
  Constant5/1 -> Switch2/3
  Constant6/1 -> Switch3/1
  Constant7/1 -> Switch3/3
  Constant8/1 -> Switch4/1
  Constant9/1 -> Switch4/3
  Constant10/1 -> Switch5/1
  Constant11/1 -> Switch5/3
  Constant12/1 -> Switch6/1
  Constant13/1 -> Switch6/3
  Constant14/1 -> Switch7/1
  Constant15/1 -> Switch7/3
  p3/1 -> Switch1/2, Switch2/2, Switch3/2, Switch4/2, Switch6/2, Switch7/2, Switch8/2, Switch9/2, Switch5/2
  Mux/1 -> Sum of Elements/1
  Sum of Elements/1 -> Multiport Switch/1
  Constant1/1 -> Mux/1
  Switch1/1 -> Mux/2
  Switch2/1 -> Mux/3
  Switch3/1 -> Mux/4
  Switch4/1 -> Mux/5
  Switch5/1 -> Mux/6
  Switch6/1 -> Mux/7
  Switch7/1 -> Mux/8
  Switch8/1 -> Mux/9
  Switch9/1 -> Mux/10
  Constant16/1 -> Switch8/1
  Constant17/1 -> Switch8/3
  Constant18/1 -> Switch9/1
  Constant19/1 -> Switch9/3
  Multiport Switch/1 -> Product/1, Product1/1
  Constant20/1 -> Multiport Switch/2
  Constant21/1 -> Multiport Switch/3
  Constant22/1 -> Multiport Switch/4
  Constant23/1 -> Multiport Switch/5
  Constant24/1 -> Multiport Switch/6
  Constant25/1 -> Multiport Switch/7
  Constant26/1 -> Multiport Switch/8
  Constant27/1 -> Multiport Switch/9
  Constant28/1 -> Multiport Switch/10
  Constant29/1 -> Multiport Switch/11
  bililiuliangfa18_1/1 -> Product/2
  bililiuliangfa18_3/1 -> Product1/2
  Product/1 -> fa18_1/1
  Product1/1 -> fa18_3/1

== system zzz/Subsystem2/shoudong/Subsystem2/Signal Builder ==
  Demux : Demux  Tag=STV Demux  Outputs=1
  FromWs : FromWorkspace  Tag=STV FromWs  VariableName=tuvar  SampleTime=0
      SigBuilderData=|
      | common.afterFinalStr = 'Extrapolate'
      | common.sampleTime = 0
      | dataSet.timeRange = [0 10]
      | dataSet.name = 'Group 1'
      | sbobj.Groups.Name = 'Group 1'
      | sbobj.Groups.Signals.Name = 'Signal 1'
      | sbobj.Groups.Signals.XData = [0 4 4 6 6 10]
      | sbobj.Groups.Signals.YData = [0 0 1 1 0 0]
  Signal 1 : Outport  Tag=STV Outport
  wires:
  FromWs/1 -> Demux/1
  Demux/1 -> Signal 1/1

== system zzz/Subsystem2/shoudong/Subsystem2/Signal Builder1 ==
  Demux : Demux  Tag=STV Demux  Outputs=1
  FromWs : FromWorkspace  Tag=STV FromWs  VariableName=tuvar  SampleTime=0
      SigBuilderData=|
      | common.afterFinalStr = 'Extrapolate'
      | common.sampleTime = 0
      | dataSet.timeRange = [0 10]
      | dataSet.name = 'Group 1'
      | sbobj.Groups.Name = 'Group 1'
      | sbobj.Groups.Signals.Name = 'Signal 1'
      | sbobj.Groups.Signals.XData = [0 4 4 6 6 10]
      | sbobj.Groups.Signals.YData = [0 0 1 1 0 0]
  Signal 1 : Outport  Tag=STV Outport
  wires:
  Demux/1 -> Signal 1/1
  FromWs/1 -> Demux/1

== system zzz/Subsystem2/shoudong/Subsystem2/Signal Builder2 ==
  Demux : Demux  Tag=STV Demux  Outputs=1
  FromWs : FromWorkspace  Tag=STV FromWs  VariableName=tuvar  SampleTime=0
      SigBuilderData=|
      | common.afterFinalStr = 'Extrapolate'
      | common.sampleTime = 0
      | dataSet.timeRange = [0 10]
      | dataSet.name = 'Group 1'
      | sbobj.Groups.Name = 'Group 1'
      | sbobj.Groups.Signals.Name = 'Signal 1'
      | sbobj.Groups.Signals.XData = [0 4 4 6 6 10]
      | sbobj.Groups.Signals.YData = [0 0 1 1 0 0]
  Signal 1 : Outport  Tag=STV Outport
  wires:
  Demux/1 -> Signal 1/1
  FromWs/1 -> Demux/1

== system zzz/Subsystem2/shoudong/Subsystem2/Signal Builder3 ==
  Demux : Demux  Tag=STV Demux  Outputs=1
  FromWs : FromWorkspace  Tag=STV FromWs  VariableName=tuvar  SampleTime=0
      SigBuilderData=|
      | common.afterFinalStr = 'Extrapolate'
      | common.sampleTime = 0
      | dataSet.timeRange = [0 10]
      | dataSet.name = 'Group 1'
      | sbobj.Groups.Name = 'Group 1'
      | sbobj.Groups.Signals.Name = 'Signal 1'
      | sbobj.Groups.Signals.XData = [0 4 4 6 6 10]
      | sbobj.Groups.Signals.YData = [0 0 1 1 0 0]
  Signal 1 : Outport  Tag=STV Outport
  wires:
  FromWs/1 -> Demux/1
  Demux/1 -> Signal 1/1

== system zzz/Subsystem2/zidong/Subsystem1/Signal Builder ==
  Demux : Demux  Tag=STV Demux  Outputs=1
  FromWs : FromWorkspace  Tag=STV FromWs  VariableName=tuvar  SampleTime=0
      SigBuilderData=|
      | common.afterFinalStr = 'Extrapolate'
      | common.sampleTime = 0
      | dataSet.timeRange = [0 10]
      | dataSet.name = 'Group 1'
      | sbobj.Groups.Name = 'Group 1'
      | sbobj.Groups.Signals.Name = 'Signal 1'
      | sbobj.Groups.Signals.XData = [0 4 4 6 6 10]
      | sbobj.Groups.Signals.YData = [0 0 1 1 0 0]
  Signal 1 : Outport  Tag=STV Outport
  wires:
  FromWs/1 -> Demux/1
  Demux/1 -> Signal 1/1

== system zzz/Subsystem2/zidong/Subsystem1/Signal Builder1 ==
  Demux : Demux  Tag=STV Demux  Outputs=1
  FromWs : FromWorkspace  Tag=STV FromWs  VariableName=tuvar  SampleTime=0
      SigBuilderData=|
      | common.afterFinalStr = 'Extrapolate'
      | common.sampleTime = 0
      | dataSet.timeRange = [0 10]
      | dataSet.name = 'Group 1'
      | sbobj.Groups.Name = 'Group 1'
      | sbobj.Groups.Signals.Name = 'Signal 1'
      | sbobj.Groups.Signals.XData = [0 4 4 6 6 10]
      | sbobj.Groups.Signals.YData = [0 0 1 1 0 0]
  Signal 1 : Outport  Tag=STV Outport
  wires:
  Demux/1 -> Signal 1/1
  FromWs/1 -> Demux/1

== system zzz/Subsystem2/zidong/Subsystem1/Signal Builder2 ==
  Demux : Demux  Tag=STV Demux  Outputs=1
  FromWs : FromWorkspace  Tag=STV FromWs  VariableName=tuvar  SampleTime=0
      SigBuilderData=|
      | common.afterFinalStr = 'Extrapolate'
      | common.sampleTime = 0
      | dataSet.timeRange = [0 10]
      | dataSet.name = 'Group 1'
      | sbobj.Groups.Name = 'Group 1'
      | sbobj.Groups.Signals.Name = 'Signal 1'
      | sbobj.Groups.Signals.XData = [0 4 4 6 6 10]
      | sbobj.Groups.Signals.YData = [0 0 1 1 0 0]
  Signal 1 : Outport  Tag=STV Outport
  wires:
  Demux/1 -> Signal 1/1
  FromWs/1 -> Demux/1

== system zzz/Subsystem2/zidong/Subsystem1/Signal Builder3 ==
  Demux : Demux  Tag=STV Demux  Outputs=1
  FromWs : FromWorkspace  Tag=STV FromWs  VariableName=tuvar  SampleTime=0
      SigBuilderData=|
      | common.afterFinalStr = 'Extrapolate'
      | common.sampleTime = 0
      | dataSet.timeRange = [0 10]
      | dataSet.name = 'Group 1'
      | sbobj.Groups.Name = 'Group 1'
      | sbobj.Groups.Signals.Name = 'Signal 1'
      | sbobj.Groups.Signals.XData = [0 4 4 6 6 10]
      | sbobj.Groups.Signals.YData = [0 0 1 1 0 0]
  Signal 1 : Outport  Tag=STV Outport
  wires:
  FromWs/1 -> Demux/1
  Demux/1 -> Signal 1/1
